simulink library "library"  (R2020a)
settings: Solver=VariableStepAuto  StartTime=0.0  StopTime=10.0  RelTol=1e-3
values from neighbouring files (symbols this model uses):
  height = 1080    [setup.m]    (also in setupSystem.m = heightName(nameIdx))
  nRho = maxRho*2    [setup.m]    (also in setupSystem.m)
  theta = (0:dTheta:180-dTheta)    [ARLHT.m]    (also in setup.m = (0:1:179); setupSystem.m = (0:1:179))
  width = 1920    [setup.m]    (also in setupSystem.m = widthName(nameIdx))
libraries: simulink x135, hdlsllib x83, $bdroot x15
(part 2 of 3)

== system library/RBM Circuit/Accumulator Memory ==
  Mode : Inport
  Address : Inport  Port=2
  Enable : Inport  Port=3
  simple_block_ram : Subsystem  VariantControl=other_bits  mask{b=1, d=nRho*nTheta, b_hidden=36, d_hidden=264600}
      mask prompts: b "Data width:"; d "Depth:"
      mask init:
      | if d == d_hidden
      |     return
      | end
      | 
      | set_param(gcb, 'd_hidden', int2str(d));
      | 
      | % Xilinx RAM Initialisation
      | xl_config = [512, 72;
      |             1024, 36;
      |             2048, 18;
      |             4096, 9;
      |             8192, 4;
      |             16384, 2;
      |             32768, 1];
      | 
      | % Get length of Xilinx Configuration
      | sizeram = size(xl_config);
      |         
      | % Get the RAM Configuration based on the data width
      | for i = 1:sizeram(1)
      |     if b <= xl_config(i, 2)
      |         a = xl_config(i, :);
      |     end
      | end
      | 
      | % Get number of BRAM required (including half BRAM)
      | numbram = ceil((d/a(1))/0.5)*0.5;
      | fullbram = floor(numbram); % Integer
      | halfbram = (numbram-floor(numbram)) ~= 0; % Boolean
      | 
      | % Get all blocks and delete everything excepts ports
      | H = get(find_system(gcb, 'FindAll', 'on', 'type', 'block'));
      | todelete = setdiff(strcat(repmat({[gcb '/']}, numel(H.Blocks), 1),  H.Blocks),...
      |     strcat(repmat({[gcb '/']}, 5, 1),...
      |     {'wr_data'; 'wr_addr'; 'wr_en'; 'rd_addr'; 'rd_data'}));
      | delete_block(todelete);
      | 
      | % Delete lines
      | for i = 1:numel(H.Lines)
      |     delete_line(H.Lines(i).Handle)
      | end
      | 
      | % Generate full BRAMs
      | y = 0;
      | 
      | % If there is only one ram then the write enable should be directly
      | % connected to the first ram write enable. Else, the write address must be sliced
      | % and the upper bound (over a(2)) compared to zero. This will indicate if
      | % the first ram is the one to be written/read from.
      | 
      | % Common to both implementations
      | % Write Address Slice
      | add_block('hdlsllib/Logic and Bit Operations/Bit Slice',...
      |         [gcb, '/wr_address'], 'Position',...
      |         [160 130 250 170]);
      | % Set bitslice parameters
      | set_param([gcb, '/wr_address'],...
      |     'lidx', int2str(log2(a(1))-1));
      | set_param([gcb, '/wr_address'],...
      |     'ridx', int2str(0));
      | 
      | % Read Address Slice
      | add_block('hdlsllib/Logic and Bit Operations/Bit Slice',...
      |         [gcb, '/rd_address'], 'Position',...
      |         [160 330 250 370]);
      | % Set bitslice parameters
      | set_param([gcb, '/rd_address'],...
      |     'lidx', int2str(log2(a(1))-1));
      | set_param([gcb, '/rd_address'],...
      |     'ridx', int2str(0));
      | 
      | if ceil(numbram) == 1
      |     
      |     i = 1;
      |     
      |     % Set bitslice parameters
      |     set_param([gcb, '/rd_address'],...
      |         'lidx', int2str(ceil(log2(d))-1));
      |     set_param([gcb, '/wr_address'],...
      |         'lidx', int2str(ceil(log2(d))-1));
      |     
      |     % Add Simple RAM
      |     add_block('hdlsllib/HDL RAMs/Simple Dual Port RAM',...
      |         [gcb, '/simple_ram_', int2str(i-1)], 'Position',...
      |         [635 0+600*y 635+200 400+600*y]);
      | 
      |     % Set RAM parameters
      |     set_param([gcb, '/simple_ram_', int2str(i-1)],...
      |         'ram_size', int2str(ceil(log2(d))));
      | 
      |     % Connect "wr_data" to "simple_ram_i"
      |     add_line(gcb, ['wr_data/1'], ['simple_ram_', int2str(i-1), '/1'],...
      |         'autorouting', 'on');
      |     
      |     % Connect "wr_addr" to "wr_address"
      |     add_line(gcb, ['wr_addr/1'], ['wr_address/1'],...
      |         'autorouting', 'on');
      | 
      |     % Connect "wr_address" to "simple_ram_i"
      |     add_line(gcb, ['wr_address/1'], ['simple_ram_', int2str(i-1), '/2'],...
      |         'autorouting', 'on');
      | 
      |     % Connect "wr_en" to "simple_ram_i"
      |     add_line(gcb, ['wr_en/1'], ['simple_ram_', int2str(i-1), '/3'],...
      |         'autorouting', 'on');
      |     
      |     % Connect "rd_addr" to "rd_address"
      |     add_line(gcb, ['rd_addr/1'], ['rd_address/1'],...
      |         'autorouting', 'on');
      | 
      |     % Connect "rd_address" to "simple_ram_i"
      |     add_line(gcb, ['rd_address/1'], ['simple_ram_', int2str(i-1), '/4'],...
      |         'autorouting', 'on');
      |     
      |     % Connect "simple_ram_i" to "rd_data"
      |     add_line(gcb, ['simple_ram_', int2str(i-1), '/1'], ['rd_data/1'],...
      |         'autorouting', 'on');
      | 
      | else
      |     
      |     % Multiport Switch
      |     add_block('hdlsllib/Signal Routing/Multiport Switch',...
      |         [gcb, '/multiport_switch'], 'Position',...
      |         [1340 146 1405 250]);
      |     % Set multiport switch parameters
      |     set_param([gcb, '/multiport_switch'],...
      |         'Inputs', int2str(ceil(numbram)));
      |     set_param([gcb, '/multiport_switch'],...
      |         'DataPortOrder', 'Zero-based contiguous');
      | 
      |     % Add Constant Zero
      |     add_block('hdlsllib/Sources/Constant',...
      |         [gcb, '/zero'], 'Position',...
      |         [425 -65 455 -35]);
      |     set_param([gcb, '/zero'],...
      |         'Value', int2str(0));
      |     set_param([gcb, '/zero'],...
      |         'OutDataTypeStr', ['fixdt(0, ', int2str(ceil(numbram)), ', 0)']);
      | 
      |     % Add Vector Concatenate
      |     add_block('hdlsllib/Signal Routing/Vector Concatenate',...
      |         [gcb, '/vector_concatenate'], 'Position',...
      |         [1015, -113, 1025, 38]);
      |     set_param([gcb, '/vector_concatenate'],...
      |         'NumInputs', int2str(ceil(numbram)));
      | 
      |     % Add Bitwise-OR
      |     add_block('hdlsllib/Logic and Bit Operations/Bitwise Operator',...
      |         [gcb, '/bitwise_or'], 'Position',...
      |         [1165, -54, 1205, -16]);
      |     set_param([gcb, '/bitwise_or'],...
      |         'logicop', 'OR');
      |     set_param([gcb, '/bitwise_or'],...
      |         'UseBitMask', 0);
      |     set_param([gcb, '/bitwise_or'],...
      |         'NumInputPorts', int2str(1));
      | 
      |     % Add delay for bram access
      |     add_block('hdlsllib/Discrete/Delay',...
      |         [gcb, '/delay'], 'Position',...
      |         [1248, 60, 1282, 95]);
      |     set_param([gcb, '/delay'],...
      |         'DelayLength', int2str(1));
      |     
      |     % Add bitslice
      |     add_block('hdlsllib/Logic and Bit Operations/Bit Slice',...
      |         [gcb, '/wr_bitslice'], 'Position',...
      |         [-65 180 25 220]);
      | 
      |     % Set bitslice parameters
      |     set_param([gcb, '/wr_bitslice'],...
      |         'lidx', int2str(ceil(log2(d)-1)));
      |     set_param([gcb, '/wr_bitslice'],...
      |         'ridx', int2str(log2(a(1))));
      |     
      |     % Add bitslice
      |     add_block('hdlsllib/Logic and Bit Operations/Bit Slice',...
      |         [gcb, '/rd_bitslice'], 'Position',...
      |         [-65 280 25 320]);
      | 
      |     % Set bitslice parameters
      |     set_param([gcb, '/rd_bitslice'],...
      |         'lidx', int2str(ceil(log2(d)-1)));
      |     set_param([gcb, '/rd_bitslice'],...
      |         'ridx', int2str(log2(a(1))));
      |     
      |     for i = 1:ceil(numbram)
      |         
      |         %%%%% Begin Adding Blocks %%%%%
      |         % Add Simple RAM
      |         add_block('hdlsllib/HDL RAMs/Simple Dual Port RAM',...
      |             [gcb, '/simple_ram_', int2str(i-1)], 'Position',...
      |             [635 0+600*y 635+200 400+600*y]);
      | 
      |         % Set RAM parameters
      |         set_param([gcb, '/simple_ram_', int2str(i-1)],...
      |             'ram_size', int2str(log2(a(1))));
      | 
      |         % Add compare to constant
      |         add_block('hdlsllib/Logic and Bit Operations/Compare To Constant',...
      |             [gcb, '/wr_cmp2const_', int2str(i-1)], 'Position',...
      |             [190 225+y*600 220 255+y*600]); 
      | 
      |         % Set compare to zero parameters
      |         set_param([gcb, '/wr_cmp2const_', int2str(i-1)],...
      |             'relop', '==');
      | 
      |         % Set compare to zero parameters
      |         set_param([gcb, '/wr_cmp2const_', int2str(i-1)],...
      |             'const', int2str(i-1));
      |         
      |         % Add compare to constant
      |         add_block('hdlsllib/Logic and Bit Operations/Compare To Constant',...
      |             [gcb, '/rd_cmp2const_', int2str(i-1)], 'Position',...
      |             [190 445+y*600 220 475+y*600]); 
      | 
      |         % Set compare to zero parameters
      |         set_param([gcb, '/rd_cmp2const_', int2str(i-1)],...
      |             'relop', '==');
      | 
      |         % Set compare to zero parameters
      |         set_param([gcb, '/rd_cmp2const_', int2str(i-1)],...
      |             'const', int2str(i-1));
      | 
      |         % Add and logic
      |         add_block('hdlsllib/Logic and Bit Operations/Logical Operator',...
      |             [gcb, '/and_', int2str(i-1)], 'Position',...
      |             [420 231+600*y 455 264+600*y]);
      | 
      |         % Set and logic parameters
      |         set_param([gcb, '/and_', int2str(i-1)],...
      |             'Operator', 'AND');
      | 
      |         % Add Switch
      |         add_block('hdlsllib/Signal Routing/Switch',...
      |             [gcb, '/switch_', int2str(i-1)], 'Position',...
      |             [685 -113+600*y 785 -37+600*y]);
      | 
      |         % Set switch parameters
      |         set_param([gcb, '/switch_', int2str(i-1)],...
      |             'Threshold', int2str(1));
      | 
      |         % Add Constant
      |         add_block('hdlsllib/Sources/Constant',...
      |             [gcb, '/constant_', int2str(i-1)], 'Position',...
      |             [425 -115+600*y 455 -85+600*y]);
      | 
      |         % Set Constant parameters
      |         set_param([gcb, '/constant_', int2str(i-1)],...
      |             'Value', int2str(i-1));
      |         set_param([gcb, '/constant_', int2str(i-1)],...
      |             'OutDataTypeStr', ['fixdt(0, ', int2str(ceil(numbram)), ', 0)']);   
      | 
      |         %%%%% Begin Wire Connections %%%%%        
      |         % Connect "wr_data" to "simple_ram_i"
      |         add_line(gcb, 'wr_data/1', ['simple_ram_', int2str(i-1), '/1'],...
      |             'autorouting','on');
      | 
      |         % Connect "wr_address" to "simple_ram_i"
      |         add_line(gcb, 'wr_address/1', ['simple_ram_', int2str(i-1), '/2'],...
      |             'autorouting','on');
      | 
      |         % Connect "rd_address" to "simple_ram_i"
      |         add_line(gcb, 'rd_address/1', ['simple_ram_', int2str(i-1), '/4'],...
      |             'autorouting','on');
      | 
      |         % Connect "constant_i" to "switch_i"
      |         add_line(gcb, ['constant_', int2str(i-1), '/1'], ['switch_', int2str(i-1), '/1'],...
      |             'autorouting','on');
      | 
      |         % Connect "zero" to "switch_i"
      |         add_line(gcb, 'zero/1', ['switch_', int2str(i-1), '/3'],...
      |             'autorouting','on');
      | 
      |         % Connect "switch_i" to "vector_concatenate"
      |         add_line(gcb, ['switch_', int2str(i-1), '/1'], ['vector_concatenate/', int2str(i)],...
      |             'autorouting','on');
      | 
      |         % Connect "rd_address" to "simple_ram_i"
      |         add_line(gcb, ['simple_ram_', int2str(i-1), '/1'], ['multiport_switch/', int2str(i+1)],...
      |             'autorouting','on');
      | 
      |         % Connect "bitslice_i" to "wr_cmp2const_i"
      |         add_line(gcb, ['wr_bitslice/1'], ['wr_cmp2const_', int2str(i-1), '/1'],...
      |             'autorouting','on');
      |         
      |         % Connect "bitslice_i" to "rd_cmp2const_i"
      |         add_line(gcb, ['rd_bitslice/1'], ['rd_cmp2const_', int2str(i-1), '/1'],...
      |             'autorouting','on');
      | 
      |         % Connect "wr_en" to "and_i"
      |         add_line(gcb, ['wr_en/1'], ['and_', int2str(i-1), '/2'],...
      |             'autorouting','on');
      | 
      |         % Connect "and_i" to "simple_ram_0"
      |         add_line(gcb, ['and_', int2str(i-1), '/1'], ['simple_ram_', int2str(i-1), '/3'],...
      |             'autorouting','on');
      | 
      |         % Connect "wr_cmp2const_i" to "and_i"
      |         add_line(gcb, ['wr_cmp2const_', int2str(i-1), '/1'], ['and_', int2str(i-1), '/1'],...
      |             'autorouting','on');
      | 
      |         % Connect "rd_cmp2const_i" to "switch_i"
      |         add_line(gcb, ['rd_cmp2const_', int2str(i-1), '/1'], ['switch_', int2str(i-1), '/2'],...
      |             'autorouting','on');
      |          
      |         % Update coordinates
      |         y = y + 1;
      |         
      |     end
      |     
      |     % Connect "rd_addr" to "bitslice_i"
      |     add_line(gcb, ['rd_addr/1'], ['rd_bitslice/1'],...
      |         'autorouting','on');
      |     
      |     % Connect "wr_addr" to "bitslice_i"
      |     add_line(gcb, ['wr_addr/1'], ['wr_bitslice/1'],...
      |         'autorouting','on');
      |     
      |     % Connect "wr_addr" to "wr_address"
      |     add_line(gcb, 'wr_addr/1', ['wr_address', '/1'],...
      |         'autorouting','on');
      | 
      |     % Connect "rd_addr" to "rd_address"
      |     add_line(gcb, 'rd_addr/1', ['rd_address', '/1'],...
      |         'autorouting','on');
      | 
      |     % Connect "vector_concatenate" to "bitwise_or"
      |     add_line(gcb, ['vector_concatenate/1'], ['bitwise_or/1'],...
      |         'autorouting','on');
      | 
      |     % Connect "bitwise_or" to "delay"
      |     add_line(gcb, ['bitwise_or/1'], ['delay/1'],...
      |         'autorouting','on');
      | 
      |     % Connect "delay" to "multiport_switch"
      |     add_line(gcb, ['delay/1'], ['multiport_switch/1'],...
      |         'autorouting','on');
      | 
      |     % Connect "multiport_switch" to "rd_data"
      |     add_line(gcb, ['multiport_switch/1'], ['rd_data/1'],...
      |         'autorouting','on');
      |     
      | end
      | 
      | % If there is a half bram we must change a few parameters. Firstly, delete
      | % the write and read address lines. Then add bitslice blocks to reduce the
      | % address space in half. Connect rd_addr and wr_addr to the corresponding ports
      | % on the bram. Finally, change the address depth.
      | if halfbram
      |     
      |     if ceil(numbram) > 1
      |         
      |         % Delete lines
      |         delete_line(gcb, ['wr_address/1'], ['simple_ram_', int2str(i-1), '/2'])
      |         delete_line(gcb, ['rd_address/1'], ['simple_ram_', int2str(i-1), '/4'])
      |         
      |         % Write Address half ram Slice
      |         add_block('hdlsllib/Logic and Bit Operations/Bit Slice',...
      |                 [gcb, '/wr_address_hr'], 'Position',...
      |                 [160 130+(y-1)*600 250 170+(y-1)*600]);
      |         % Set bitslice parameters
      |         set_param([gcb, '/wr_address_hr'],...
      |             'lidx', int2str(log2(a(1))-2));
      |         set_param([gcb, '/wr_address_hr'],...
      |             'ridx', int2str(0));
      | 
      |         % Read Address half ram Slice
      |         add_block('hdlsllib/Logic and Bit Operations/Bit Slice',...
      |                 [gcb, '/rd_address_hr'], 'Position',...
      |                 [160 330+(y-1)*600 250 370+(y-1)*600]);
      |         % Set bitslice parameters
      |         set_param([gcb, '/rd_address_hr'],...
      |             'lidx', int2str(log2(a(1))-2));
      |         set_param([gcb, '/rd_address_hr'],...
      |             'ridx', int2str(0));
      | 
      |         % Connect "wr_addr" to "wr_address_hr"
      |         add_line(gcb, 'wr_addr/1', ['wr_address_hr', '/1'],...
      |             'autorouting','on');
      | 
      |         % Connect "rd_addr" to "rd_address_hr"
      |         add_line(gcb, 'rd_addr/1', ['rd_address_hr', '/1'],...
      |             'autorouting','on');
      | 
      |         % Connect "wr_address_hr" to "simple_ram_i"
      |         add_line(gcb, ['wr_address_hr', '/1'], ['simple_ram_', int2str(i-1), '/2'],...
      |             'autorouting','on');
      | 
      |         % Connect "rd_address_hr" to "simple_ram_i"
      |         add_line(gcb, ['rd_address_hr', '/1'], ['simple_ram_', int2str(i-1), '/4'],...
      |             'autorouting','on');
      |         
      |         % Update the ram parameters (address bits)
      |         set_param([gcb, '/simple_ram_', int2str(i-1)],...
      |             'ram_size', int2str(log2(a(1)/2)));
      | 
      |     else
      |         % Set bitslice parameters
      |         % set_param([gcb, '/wr_address'],...
      |         %     'lidx', int2str(log2(a(1))-2));
      |         % set_param([gcb, '/wr_address'],...
      |         %     'ridx', int2str(0));
      |         % Set bitslice parameters
      |         % set_param([gcb, '/rd_address'],...
      |         %     'lidx', int2str(log2(a(1))-2));
      |         % set_param([gcb, '/rd_address'],...
      |         %     'ridx', int2str(0));
      |         
      |     end
      |     
      | 
      |     
      | end
  RBM : Outport
  wires:
  Mode/1 -> simple_block_ram/1(wr_data)
  Enable/1 -> simple_block_ram/3(wr_en)
  Address/1 -> simple_block_ram/2(wr_addr), simple_block_ram/4(rd_addr)
  simple_block_ram/1(rd_data) -> RBM/1

== system library/Sobel Filter/Coordinate Counters ==
  Valid In : Inport
  AND : Logic  IconShape=distinctive  AllPortsSameDT=off  OutDataTypeStr=boolean
  Compare To Constant : simulink/Logic and Bit Operations/Compare To Constant  relop===  const=width/2-1  OutDataTypeStr=boolean
  X Counter : hdlsllib/Sources/HDL Counter  CountType=Count limited  CountInit=-width/2  CountStep=1  CountMax=width/2-1  CountFromType=Initial value  CountFrom=-width/2  CountResetPort=off  CountLoadPort=off  CountEnbPort=on  CountDirPort=off  CountDataType=Signed  CountWordLen=ceil(log2(width/2)) + 1  CountFracLen=0  CountSampTime=1
  Y Counter : hdlsllib/Sources/HDL Counter  CountType=Count limited  CountInit=-height/2  CountStep=1  CountMax=height/2-1  CountFromType=Initial value  CountFrom=-height/2  CountResetPort=off  CountLoadPort=off  CountEnbPort=on  CountDirPort=off  CountDataType=Signed  CountWordLen=ceil(log2(height/2)) + 1  CountFracLen=0  CountSampTime=1
  X Value : Outport  VectorParamsAs1DForOutWhenUnconnected=off
  Y Value : Outport  Port=2  VectorParamsAs1DForOutWhenUnconnected=off
  wires:
  Compare To Constant/1 -> AND/1
  AND/1 -> Y Counter/1
  Y Counter/1 -> Y Value/1
  X Counter/1 -> Compare To Constant/1, X Value/1
  Valid In/1 -> X Counter/1, AND/2

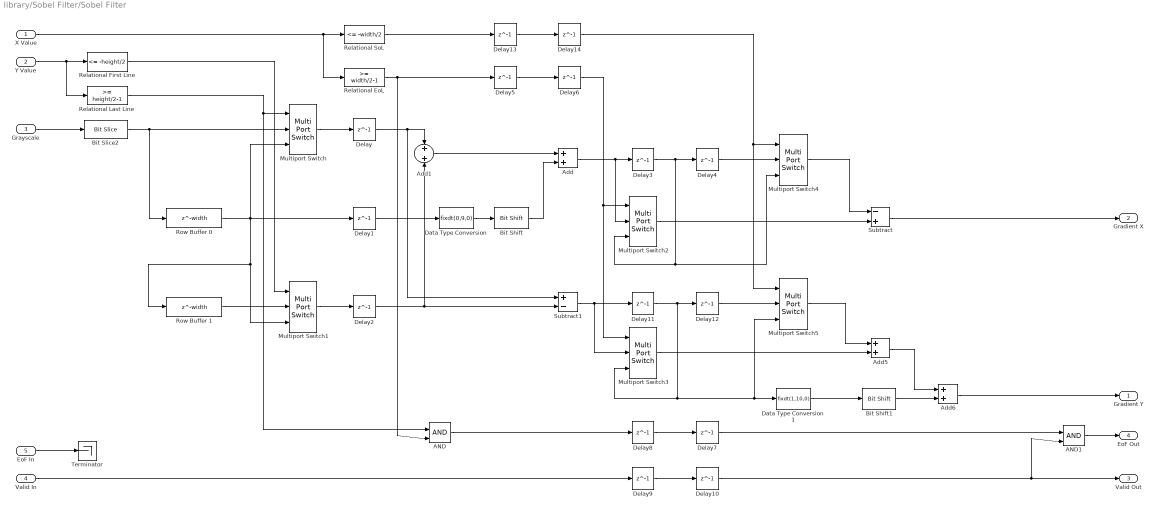
== system library/Sobel Filter/Sobel Filter ==
  X Value : Inport
  Y Value : Inport  Port=2
  Grayscale : Inport  Port=3
  Valid In : Inport  Port=4
  EoF In : Inport  Port=5
  AND : Logic  IconShape=distinctive  AllPortsSameDT=off  OutDataTypeStr=boolean
  AND1 : Logic  IconShape=distinctive  AllPortsSameDT=off  OutDataTypeStr=boolean
  Add{,1,5..6} (4 alike) : Sum
  Bit Shift : hdlsllib/Logic and Bit Operations/Bit Shift  mode=Shift Left Logical  N=1
  Bit Shift1 : hdlsllib/Logic and Bit Operations/Bit Shift  mode=Shift Left Logical  N=1
  Bit Slice2 : hdlsllib/Logic and Bit Operations/Bit Slice  lidx=7  ridx=0
      settings: SourceProductBaseCode=SL
  Data Type Conversion : DataTypeConversion  OutDataTypeStr=fixdt(0,9,0)
  Data Type Conversion1 : DataTypeConversion  OutDataTypeStr=fixdt(1,10,0)
  Delay{,1..14} (15 alike) : Delay  DelayLength=1
  Multiport Switch{,1..5} (6 alike) : MultiPortSwitch  DataPortOrder=Zero-based contiguous  Inputs=2  zeroidx=on
  Relational EoL : simulink/Logic and Bit Operations/Compare To Constant  relop=>=  const=width/2-1  OutDataTypeStr=boolean
  Relational First Line : simulink/Logic and Bit Operations/Compare To Constant  relop=<=  const=-height/2  OutDataTypeStr=boolean
  Relational Last Line : simulink/Logic and Bit Operations/Compare To Constant  relop=>=  const=height/2-1  OutDataTypeStr=boolean
  Relational SoL : simulink/Logic and Bit Operations/Compare To Constant  relop=<=  const=-width/2  OutDataTypeStr=boolean
  Row Buffer 0 : Delay  DelayLength=width
  Row Buffer 1 : Delay  DelayLength=width
  Subtract : Sum  Inputs=-+
  Subtract1 : Sum  Inputs=+-
  Terminator : Terminator
  Gradient Y : Outport
  Gradient X : Outport  Port=2
  Valid Out : Outport  Port=3
  EoF Out : Outport  Port=4
  wires:
  Data Type Conversion1/1 -> Bit Shift1/1
  Bit Shift/1 -> Add/2
  AND1/1 -> EoF Out/1
  Delay7/1 -> AND1/1
  Delay14/1 -> Multiport Switch4/1, Multiport Switch5/1
  Delay13/1 -> Delay14/1
  Relational SoL/1 -> Delay13/1
  Multiport Switch5/1 -> Add5/1
  Delay12/1 -> Multiport Switch5/2
  Multiport Switch4/1 -> Subtract/1
  Delay4/1 -> Multiport Switch4/2
  Delay6/1 -> Multiport Switch3/1, Multiport Switch2/1
  Delay5/1 -> Delay6/1
  Relational EoL/1 -> Delay5/1, AND/2
  Multiport Switch3/1 -> Add5/2
  Subtract1/1 -> Multiport Switch3/2, Delay11/1
  Add/1 -> Multiport Switch2/2, Delay3/1
  Multiport Switch2/1 -> Subtract/2
  Row Buffer 1/1 -> Multiport Switch1/2
  Row Buffer 0/1 -> Multiport Switch/3, Delay1/1, Multiport Switch1/3, Row Buffer 1/1
  Relational First Line/1 -> Multiport Switch1/1
  Multiport Switch1/1 -> Delay2/1
  Relational Last Line/1 -> Multiport Switch/1, AND/1
  Multiport Switch/1 -> Delay/1
  X Value/1 -> Relational SoL/1, Relational EoL/1
  Y Value/1 -> Relational First Line/1, Relational Last Line/1
  Bit Shift1/1 -> Add6/2
  Add5/1 -> Add6/1
  Delay11/1 -> Multiport Switch5/3, Data Type Conversion1/1, Multiport Switch3/3, Delay12/1
  Delay2/1 -> Add1/2, Subtract1/2
  Subtract/1 -> Gradient X/1
  Delay1/1 -> Data Type Conversion/1
  Add1/1 -> Add/1
  Delay/1 -> Subtract1/1, Add1/1
  Data Type Conversion/1 -> Bit Shift/1
  Delay3/1 -> Delay4/1, Multiport Switch4/3, Multiport Switch2/3
  Delay10/1 -> Valid Out/1, AND1/2
  Delay9/1 -> Delay10/1
  Valid In/1 -> Delay9/1
  AND/1 -> Delay8/1
  Delay8/1 -> Delay7/1
  Add6/1 -> Gradient Y/1
  EoF In/1 -> Terminator/1
  Bit Slice2/1 -> Row Buffer 0/1, Multiport Switch/2
  Grayscale/1 -> Bit Slice2/1

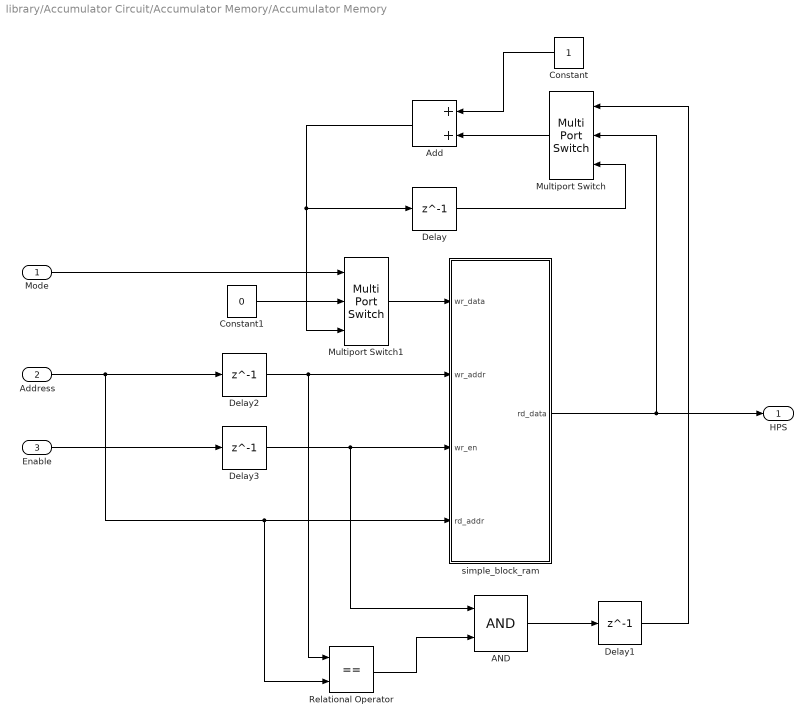
== system library/Accumulator Circuit/Accumulator Memory/Accumulator Memory ==
  Mode : Inport
  Address : Inport  Port=2
  Enable : Inport  Port=3
  AND : Logic  IconShape=distinctive  AllPortsSameDT=off  OutDataTypeStr=boolean
  Add : Sum  OutDataTypeStr=fixdt(0,rhoBits,0)
  Constant : Constant  OutDataTypeStr=fixdt(0,1,0)  SampleTime=-1
  Constant1 : Constant  Value=0  OutDataTypeStr=fixdt(0,rhoBits,0)  SampleTime=-1
  Delay{,1..3} (4 alike) : Delay  DelayLength=1
  Multiport Switch : MultiPortSwitch  DataPortOrder=Zero-based contiguous  Inputs=2  zeroidx=on
  Multiport Switch1 : MultiPortSwitch  DataPortOrder=Zero-based contiguous  Inputs=2  zeroidx=on
  Relational Operator : RelationalOperator  Operator===  OutDataTypeStr=boolean  RndMeth=Simplest
  simple_block_ram : Subsystem  VariantControl=other_bits  mask{b=rhoBits, d=nRho*nTheta/kTheta, b_hidden=36, d_hidden=99180}
      mask prompts: b "Data width:"; d "Depth:"
      mask init: same as library/RBM Circuit/Accumulator Memory/simple_block_ram
  HPS : Outport
  wires:
  Delay1/1 -> Multiport Switch/1
  Enable/1 -> Delay3/1
  Relational Operator/1 -> AND/2
  Delay3/1 -> simple_block_ram/3(wr_en), AND/1
  Add/1 -> Delay/1, Multiport Switch1/3
  Constant1/1 -> Multiport Switch1/2
  Constant/1 -> Add/1
  Delay2/1 -> simple_block_ram/2(wr_addr), Relational Operator/1
  Multiport Switch/1 -> Add/2
  Delay/1 -> Multiport Switch/3
  AND/1 -> Delay1/1
  simple_block_ram/1(rd_data) -> Multiport Switch/2, HPS/1
  Address/1 -> Delay2/1, simple_block_ram/4(rd_addr), Relational Operator/2
  Multiport Switch1/1 -> simple_block_ram/1(wr_data)
  Mode/1 -> Multiport Switch1/1

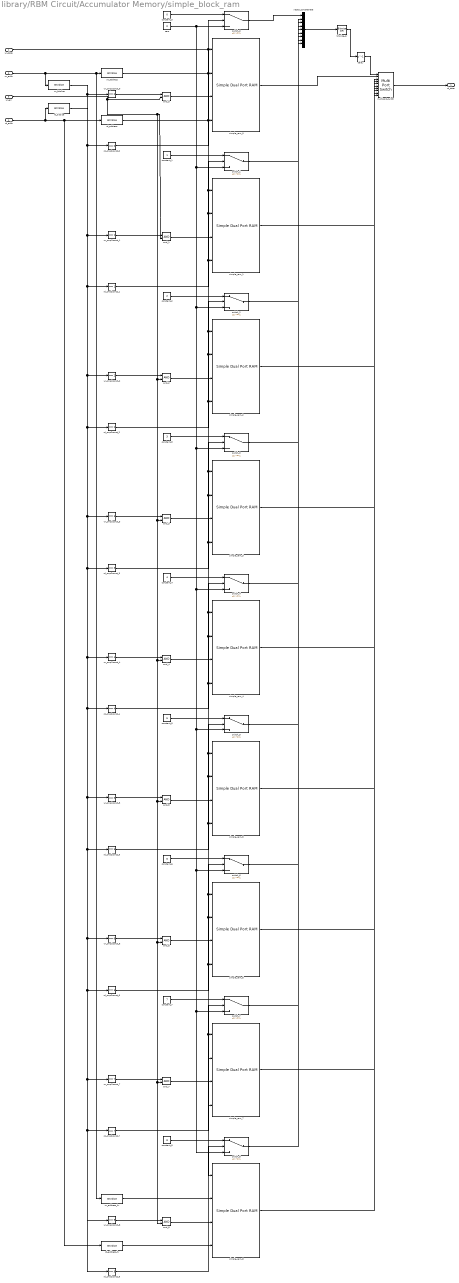
== system library/RBM Circuit/Accumulator Memory/simple_block_ram ==
  wr_data : Inport
  wr_addr : Inport  Port=2
  wr_en : Inport  Port=3
  rd_addr : Inport  Port=4
  and_{0..8} (9 alike) : Logic  AllPortsSameDT=off  OutDataTypeStr=boolean
  bitwise_or : simulink/Logic and Bit Operations/Bitwise Operator  logicop=OR  UseBitMask=off  BitMask=bin2dec('11011001')  BitMaskRealWorld=Stored Integer
  constant_0 : Constant  Value=0  OutDataTypeStr=fixdt(0, 9, 0)  SampleTime=-1
  constant_1 : Constant  OutDataTypeStr=fixdt(0, 9, 0)  SampleTime=-1
  constant_2 : Constant  Value=2  OutDataTypeStr=fixdt(0, 9, 0)  SampleTime=-1
  constant_3 : Constant  Value=3  OutDataTypeStr=fixdt(0, 9, 0)  SampleTime=-1
  constant_4 : Constant  Value=4  OutDataTypeStr=fixdt(0, 9, 0)  SampleTime=-1
  constant_5 : Constant  Value=5  OutDataTypeStr=fixdt(0, 9, 0)  SampleTime=-1
  constant_6 : Constant  Value=6  OutDataTypeStr=fixdt(0, 9, 0)  SampleTime=-1
  constant_7 : Constant  Value=7  OutDataTypeStr=fixdt(0, 9, 0)  SampleTime=-1
  constant_8 : Constant  Value=8  OutDataTypeStr=fixdt(0, 9, 0)  SampleTime=-1
  delay : Delay  DelayLength=1
  multiport_switch : MultiPortSwitch  DataPortOrder=Zero-based contiguous  Inputs=9  zeroidx=on
  rd_address : hdlsllib/Logic and Bit Operations/Bit Slice  lidx=14  ridx=0
      settings: SourceProductBaseCode=SL
  rd_address_hr : hdlsllib/Logic and Bit Operations/Bit Slice  lidx=13  ridx=0
      settings: SourceProductBaseCode=SL
  rd_bitslice : hdlsllib/Logic and Bit Operations/Bit Slice  lidx=18  ridx=15
      settings: SourceProductBaseCode=SL
  rd_cmp2const_0 : simulink/Logic and Bit Operations/Compare To Constant  relop===  const=0  OutDataTypeStr=boolean
  rd_cmp2const_1 : simulink/Logic and Bit Operations/Compare To Constant  relop===  const=1  OutDataTypeStr=boolean
  rd_cmp2const_2 : simulink/Logic and Bit Operations/Compare To Constant  relop===  const=2  OutDataTypeStr=boolean
  rd_cmp2const_3 : simulink/Logic and Bit Operations/Compare To Constant  relop===  const=3  OutDataTypeStr=boolean
  rd_cmp2const_4 : simulink/Logic and Bit Operations/Compare To Constant  relop===  const=4  OutDataTypeStr=boolean
  rd_cmp2const_5 : simulink/Logic and Bit Operations/Compare To Constant  relop===  const=5  OutDataTypeStr=boolean
  rd_cmp2const_6 : simulink/Logic and Bit Operations/Compare To Constant  relop===  const=6  OutDataTypeStr=boolean
  rd_cmp2const_7 : simulink/Logic and Bit Operations/Compare To Constant  relop===  const=7  OutDataTypeStr=boolean
  rd_cmp2const_8 : simulink/Logic and Bit Operations/Compare To Constant  relop===  const=8  OutDataTypeStr=boolean
  simple_ram_{0..7} (8 alike) : hdlsllib/HDL RAMs/Simple Dual Port RAM  ram_size=15
      settings: SourceProductBaseCode=SL
  simple_ram_8 : hdlsllib/HDL RAMs/Simple Dual Port RAM  ram_size=14
      settings: SourceProductBaseCode=SL
  switch_{0..8} (9 alike) : Switch  Threshold=1
  vector_concatenate : Concatenate  NumInputs=9
  wr_address : hdlsllib/Logic and Bit Operations/Bit Slice  lidx=14  ridx=0
      settings: SourceProductBaseCode=SL
  wr_address_hr : hdlsllib/Logic and Bit Operations/Bit Slice  lidx=13  ridx=0
      settings: SourceProductBaseCode=SL
  wr_bitslice : hdlsllib/Logic and Bit Operations/Bit Slice  lidx=18  ridx=15
      settings: SourceProductBaseCode=SL
  wr_cmp2const_0 : simulink/Logic and Bit Operations/Compare To Constant  relop===  const=0  OutDataTypeStr=boolean
  wr_cmp2const_1 : simulink/Logic and Bit Operations/Compare To Constant  relop===  const=1  OutDataTypeStr=boolean
  wr_cmp2const_2 : simulink/Logic and Bit Operations/Compare To Constant  relop===  const=2  OutDataTypeStr=boolean
  wr_cmp2const_3 : simulink/Logic and Bit Operations/Compare To Constant  relop===  const=3  OutDataTypeStr=boolean
  wr_cmp2const_4 : simulink/Logic and Bit Operations/Compare To Constant  relop===  const=4  OutDataTypeStr=boolean
  wr_cmp2const_5 : simulink/Logic and Bit Operations/Compare To Constant  relop===  const=5  OutDataTypeStr=boolean
  wr_cmp2const_6 : simulink/Logic and Bit Operations/Compare To Constant  relop===  const=6  OutDataTypeStr=boolean
  wr_cmp2const_7 : simulink/Logic and Bit Operations/Compare To Constant  relop===  const=7  OutDataTypeStr=boolean
  wr_cmp2const_8 : simulink/Logic and Bit Operations/Compare To Constant  relop===  const=8  OutDataTypeStr=boolean
  zero : Constant  Value=0  OutDataTypeStr=fixdt(0, 9, 0)  SampleTime=-1
  rd_data : Outport
  wires:
  rd_address_hr/1 -> simple_ram_8/4
  wr_address_hr/1 -> simple_ram_8/2
  multiport_switch/1 -> rd_data/1
  delay/1 -> multiport_switch/1
  bitwise_or/1 -> delay/1
  vector_concatenate/1 -> bitwise_or/1
  wr_addr/1 -> wr_bitslice/1, wr_address_hr/1, wr_address/1
  rd_addr/1 -> rd_bitslice/1, rd_address_hr/1, rd_address/1
  rd_cmp2const_8/1 -> switch_8/2
  wr_cmp2const_8/1 -> and_8/1
  and_8/1 -> simple_ram_8/3
  simple_ram_8/1 -> multiport_switch/10
  switch_8/1 -> vector_concatenate/9
  constant_8/1 -> switch_8/1
  rd_cmp2const_7/1 -> switch_7/2
  wr_cmp2const_7/1 -> and_7/1
  and_7/1 -> simple_ram_7/3
  simple_ram_7/1 -> multiport_switch/9
  switch_7/1 -> vector_concatenate/8
  constant_7/1 -> switch_7/1
  rd_cmp2const_6/1 -> switch_6/2
  wr_cmp2const_6/1 -> and_6/1
  and_6/1 -> simple_ram_6/3
  simple_ram_6/1 -> multiport_switch/8
  switch_6/1 -> vector_concatenate/7
  constant_6/1 -> switch_6/1
  rd_cmp2const_5/1 -> switch_5/2
  wr_cmp2const_5/1 -> and_5/1
  and_5/1 -> simple_ram_5/3
  simple_ram_5/1 -> multiport_switch/7
  switch_5/1 -> vector_concatenate/6
  constant_5/1 -> switch_5/1
  rd_cmp2const_4/1 -> switch_4/2
  wr_cmp2const_4/1 -> and_4/1
  and_4/1 -> simple_ram_4/3
  simple_ram_4/1 -> multiport_switch/6
  switch_4/1 -> vector_concatenate/5
  constant_4/1 -> switch_4/1
  rd_cmp2const_3/1 -> switch_3/2
  wr_cmp2const_3/1 -> and_3/1
  and_3/1 -> simple_ram_3/3
  simple_ram_3/1 -> multiport_switch/5
  switch_3/1 -> vector_concatenate/4
  constant_3/1 -> switch_3/1
  rd_cmp2const_2/1 -> switch_2/2
  wr_cmp2const_2/1 -> and_2/1
  and_2/1 -> simple_ram_2/3
  simple_ram_2/1 -> multiport_switch/4
  switch_2/1 -> vector_concatenate/3
  constant_2/1 -> switch_2/1
  rd_cmp2const_1/1 -> switch_1/2
  wr_cmp2const_1/1 -> and_1/1
  and_1/1 -> simple_ram_1/3
  simple_ram_1/1 -> multiport_switch/3
  switch_1/1 -> vector_concatenate/2
  constant_1/1 -> switch_1/1
  rd_cmp2const_0/1 -> switch_0/2
  wr_cmp2const_0/1 -> and_0/1
  and_0/1 -> simple_ram_0/3
  wr_en/1 -> and_0/2, and_1/2, and_2/2, and_3/2, and_4/2, and_5/2, and_6/2, and_8/2, and_7/2
  rd_bitslice/1 -> rd_cmp2const_0/1, rd_cmp2const_1/1, rd_cmp2const_2/1, rd_cmp2const_3/1, rd_cmp2const_4/1, rd_cmp2const_5/1, rd_cmp2const_6/1, rd_cmp2const_8/1, rd_cmp2const_7/1
  wr_bitslice/1 -> wr_cmp2const_0/1, wr_cmp2const_1/1, wr_cmp2const_2/1, wr_cmp2const_3/1, wr_cmp2const_4/1, wr_cmp2const_5/1, wr_cmp2const_6/1, wr_cmp2const_8/1, wr_cmp2const_7/1
  simple_ram_0/1 -> multiport_switch/2
  switch_0/1 -> vector_concatenate/1
  zero/1 -> switch_0/3, switch_1/3, switch_2/3, switch_3/3, switch_4/3, switch_5/3, switch_6/3, switch_8/3, switch_7/3
  constant_0/1 -> switch_0/1
  rd_address/1 -> simple_ram_0/4, simple_ram_1/4, simple_ram_2/4, simple_ram_3/4, simple_ram_4/4, simple_ram_5/4, simple_ram_7/4, simple_ram_6/4
  wr_address/1 -> simple_ram_0/2, simple_ram_1/2, simple_ram_2/2, simple_ram_3/2, simple_ram_4/2, simple_ram_5/2, simple_ram_7/2, simple_ram_6/2
  wr_data/1 -> simple_ram_0/1, simple_ram_1/1, simple_ram_2/1, simple_ram_3/1, simple_ram_4/1, simple_ram_5/1, simple_ram_6/1, simple_ram_8/1, simple_ram_7/1
